simulink model "multivar_output"  (Simulink 7.3)
settings: Solver=ode45  StartTime=0.0  StopTime=10.0  RelTol=1e-3
undefined symbols (not defined in the file or in its folder): sizeyunsuan
settings Model: Creator=sn00632  LastModifiedBy=sn00632

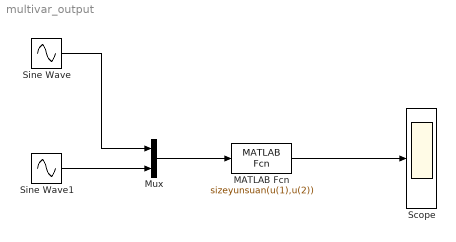
== system multivar_output ==
  MATLAB Fcn : MATLABFcn  MATLABFcn=sizeyunsuan(u(1),u(2))  OutputDimensions=5  Output1D=off
  Mux : Mux  Inputs=2
  Scope : Scope
  Sine Wave : Sin  Amplitude=1  Bias=0  Frequency=1  Phase=0  Samples=10  SampleTime=0  Offset=0
  Sine Wave1 : Sin  Amplitude=1  Bias=0  Frequency=1  Phase=0  Samples=10  SampleTime=0  Offset=0
  wires:
  Sine Wave/1 -> Mux/1
  Sine Wave1/1 -> Mux/2
  Mux/1 -> MATLAB Fcn/1
  MATLAB Fcn/1 -> Scope/1
